simulink model "Lorentz_Equations"  (Simulink 10.0)
settings: Solver=ode45  StartTime=0.0  StopTime=300  MaxStep=0.1  MinStep=0.01  RelTol=1e-6
settings Model: Creator=szymo  LastModifiedBy=szymo
settings DataIOCC: SaveFormat=Dataset  ReturnWorkspaceOutputs=on
settings OptimizationCC: LifeSpan=auto
settings DebuggingCC: UnderspecifiedInitializationDetection=Simplified  MergeDetectMultiDrivingBlocksExec=error  SFUnexpectedBacktrackingDiag=error  SFNoUnconditionalDefaultTransitionDiag=error  SFExecutionAtInitializationDiag=warning  ArithmeticOperatorsInVariantConditions=error
settings HardwareCC: ProdBitPerPointer=64  ProdBitPerSizeT=64  ProdBitPerPtrDiffT=64  ProdLargestAtomicFloat=Float  ProdIntDivRoundTo=Zero  ProdEndianess=LittleEndian  ProdWordSize=64  ProdHWDeviceType=Intel->x86-64 (Windows64)
settings ModelReferenceCC: PropagateSignalLabelsOutOfModel=on
settings SFSimCC: SimUseLocalCustomCode=on  CustomCodeUndefinedFunction=FilterOut
settings RTWCC: RTWUseLocalCustomCode=on
settings CodeAppCC: StateflowObjectComments=off
settings GRTTargetCC: TargetLangStandard=C99 (ISO)  CombineOutputUpdateFcns=on  GRTInterface=off
settings ConfigComp: CovMetricSettings=dwe  CovHtmlReporting=off  CovSaveCumulativeToWorkspaceVar=off  CovSaveSingleToWorkspaceVar=off

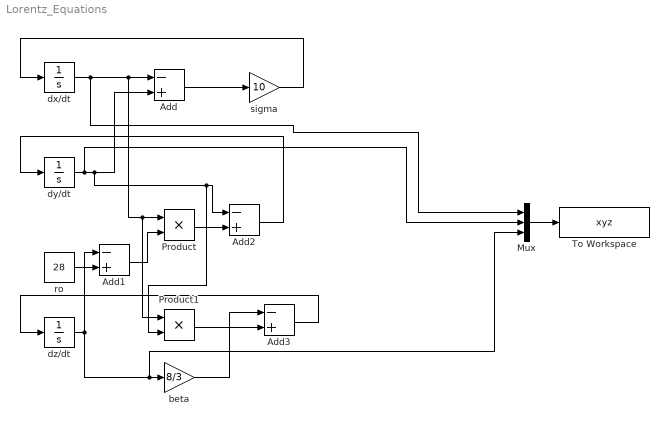
== system Lorentz_Equations ==
  Add{,1..3} (4 alike) : Sum  Inputs=-+
  Mux : Mux  Inputs=3
  Product : Product
  Product1 : Product
  To Workspace : ToWorkspace  VariableName=xyz  SaveFormat=Timeseries  SampleTime=-1
  beta : Gain  Gain=8/3
  dx/dt : Integrator  InitialCondition=0.001
  dy/dt : Integrator  InitialCondition=0.001
  dz/dt : Integrator  InitialCondition=0.001
  ro : Constant  Value=28
  sigma : Gain  Gain=10
  wires:
  dy/dt/1 -> Mux/2, Product1/2, Add2/1, Add/2
  dx/dt/1 -> Mux/1, Product1/1, Product/1, Add/1
  Add/1 -> sigma/1
  sigma/1 -> dx/dt/1
  Add1/1 -> Product/2
  ro/1 -> Add1/2
  dz/dt/1 -> Mux/3, beta/1, Add1/1
  Product/1 -> Add2/2
  Add2/1 -> dy/dt/1
  Product1/1 -> Add3/2
  beta/1 -> Add3/1
  Add3/1 -> dz/dt/1
  Mux/1 -> To Workspace/1
